simulink model "Test_Subtractor"  (Simulink 8.1)
settings: Solver=ode45  StartTime=0.0  StopTime=10.0  RelTol=1e-3
libraries: Computer_Library x2
settings Model: Creator=N  LastModifiedBy=uzivatel
settings DataIOCC: LimitDataPoints=off  SignalLoggingSaveFormat=Dataset
settings OptimizationCC: ExpressionDepthLimit=128
settings DebuggingCC: UnderspecifiedInitializationDetection=Simplified  MergeDetectMultiDrivingBlocksExec=error  SolverPrmCheckMsg=none  FcnCallInpInsideContextMsg=EnableAllAsError  FrameProcessingCompatibilityMsg=error  StateNameClashWarn=none
settings HardwareCC: ProdBitPerPointer=64  ProdLargestAtomicFloat=Float  ProdIntDivRoundTo=Zero  ProdEndianess=LittleEndian  ProdHWDeviceType=Intel->x86-64 (Windows64)
settings ModelReferenceCC: PropagateSignalLabelsOutOfModel=on
settings GRTTargetCC: CodeReplacementLibrary=None  CombineOutputUpdateFcns=on  CPPClassGenCompliant=on  GRTInterface=off

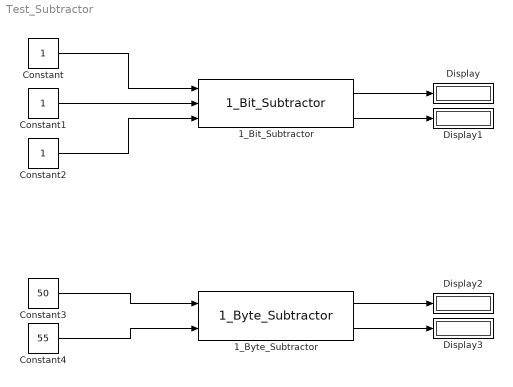
== system Test_Subtractor ==
  1_Bit_Subtractor : Computer_Library/Subtractors/1_Bit_Subtractor
  1_Byte_Subtractor : Computer_Library/Subtractors/1_Byte_Subtractor
  Constant : Constant
  Constant1 : Constant
  Constant2 : Constant
  Constant3 : Constant  Value=50
  Constant4 : Constant  Value=55
  Display{,1..3} (4 alike) : Display
  wires:
  1_Bit_Subtractor/1 -> Display/1
  1_Bit_Subtractor/2 -> Display1/1
  Constant2/1 -> 1_Bit_Subtractor/3
  Constant1/1 -> 1_Bit_Subtractor/2
  Constant/1 -> 1_Bit_Subtractor/1
  1_Byte_Subtractor/1 -> Display2/1
  1_Byte_Subtractor/2 -> Display3/1
  Constant4/1 -> 1_Byte_Subtractor/2
  Constant3/1 -> 1_Byte_Subtractor/1
